simulink model "quadrotor_control2"  (R2017b)
settings: Solver=FixedStepAuto  StartTime=0.0  StopTime=10  FixedStep=0.0001  RelTol=1e-3  EnableMultiTasking=on
PreLoadFcn:
  | m=0;
libraries: simulink x9
settings Model: Creator=GPH_PC  LastModifiedBy=dell
settings DataIOCC: LimitDataPoints=on  SaveFormat=Array
settings OptimizationCC: LifeSpan=inf
settings DebuggingCC: SolverPrmCheckMsg=warning  SFUnexpectedBacktrackingDiag=warning  SFNoUnconditionalDefaultTransitionDiag=warning  SFExecutionAtInitializationDiag=none
settings HardwareCC: ProdBitPerPointer=32  ProdBitPerSizeT=32  ProdBitPerPtrDiffT=32  ProdLargestAtomicFloat=None  ProdIntDivRoundTo=Undefined  ProdEndianess=Unspecified  ProdWordSize=32  ProdHWDeviceType=32-bit Generic
settings ModelReferenceCC: PropagateSignalLabelsOutOfModel=off
settings CodeAppCC: StateflowObjectComments=on
settings GRTTargetCC: TargetLangStandard=C89/C90 (ANSI)  GeneratePreprocessorConditionals=Disable all
settings ConfigComp: CovMetricSettings=dw  CovHtmlReporting=on  CovSaveCumulativeToWorkspaceVar=on  CovSaveSingleToWorkspaceVar=on  CovExternalEMLEnable=off  CovSFcnEnable=off

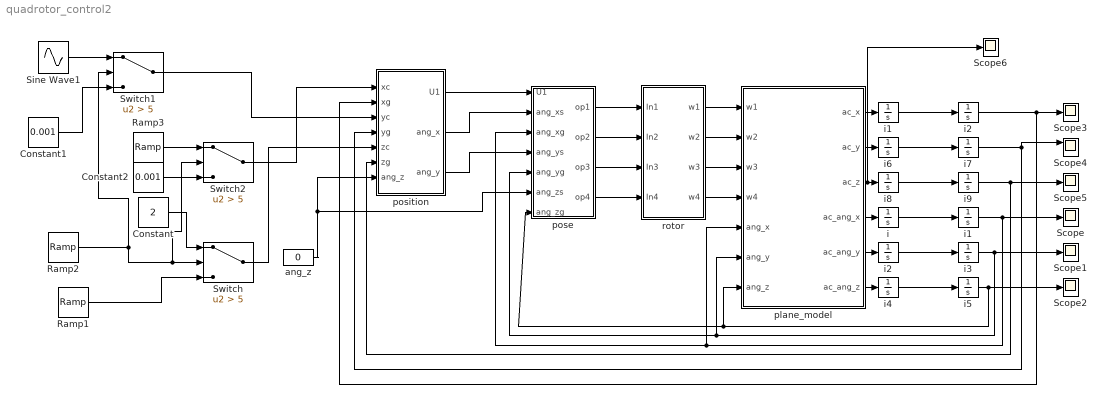
== system quadrotor_control2 ==
  " i1" : Integrator
  " i2" : Integrator
  Constant : Constant  Value=2
  Constant1 : Constant  Value=0.001
  Constant2 : Constant  Value=0.001
  Ramp1 : simulink/Sources/Ramp  slope=0.2  start=0  X0=0
  Ramp2 : simulink/Sources/Ramp  slope=1  start=0  X0=0
  Ramp3 : simulink/Sources/Ramp  slope=1  start=0  X0=0
  Scope{,1..3,5..6} (6 alike) : Scope
  Scope4 : Scope  NumInputPorts=3
  Sine Wave1 : Sin  Amplitude=3  SampleTime=0
  Switch : Switch  Criteria=u2 > Threshold  Threshold=5
  Switch1 : Switch  Criteria=u2 > Threshold  Threshold=5
  Switch2 : Switch  Criteria=u2 > Threshold  Threshold=5
  ang_z : Constant  Value=0
  i{,1..9} (10 alike) : Integrator
  plane_model : MATLAB Function  TreatAsAtomicUnit=on
  pose : Subsystem
  position : Subsystem
  rotor : Subsystem
  wires:
  rotor/1(w1) -> plane_model/1(w1)
  rotor/2(w2) -> plane_model/2(w2)
  rotor/3(w3) -> plane_model/3(w3)
  rotor/4(w4) -> plane_model/4(w4)
  pose/1(op1) -> rotor/1(In1)
  pose/2(op2) -> rotor/2(In2)
  pose/3(op3) -> rotor/3(In3)
  pose/4(op4) -> rotor/4(In4)
  plane_model/4(ac_ang_x) -> i/1
  i/1 -> " i1"/1
  i2/1 -> i3/1
  i4/1 -> i5/1
  plane_model/5(ac_ang_y) -> i2/1
  plane_model/6(ac_ang_z) -> i4/1
  i5/1 -> plane_model/7(ang_z), pose/7(ang_zg), Scope2/1
  i3/1 -> pose/5(ang_yg), plane_model/6(ang_y), Scope1/1
  " i1"/1 -> pose/3(ang_xg), plane_model/5(ang_x), Scope/1
  i1/1 -> " i2"/1
  i6/1 -> i7/1
  i8/1 -> i9/1
  plane_model/3(ac_z) -> Scope6/1, i8/1
  plane_model/2(ac_y) -> i6/1
  plane_model/1(ac_x) -> i1/1
  i9/1 -> Scope5/1, position/6(zg)
  i7/1 -> position/4(yg), Scope4/1
  position/1(U1) -> pose/1(U1)
  position/2(ang_x) -> pose/2(ang_xs)
  position/3(ang_y) -> pose/4(ang_ys)
  ang_z/1 -> position/7(ang_z), pose/6(ang_zs)
  " i2"/1 -> Scope3/1, position/2(xg)
  Constant1/1 -> Switch1/3
  Ramp2/1 -> Switch2/2, Switch/2, Switch1/2
  Constant2/1 -> Switch2/3
  Ramp3/1 -> Switch2/1
  Ramp1/1 -> Switch/3
  Constant/1 -> Switch/1
  Sine Wave1/1 -> Switch1/1
  Switch1/1 -> position/3(yc)
  Switch2/1 -> position/1(xc)
  Switch/1 -> position/5(zc)

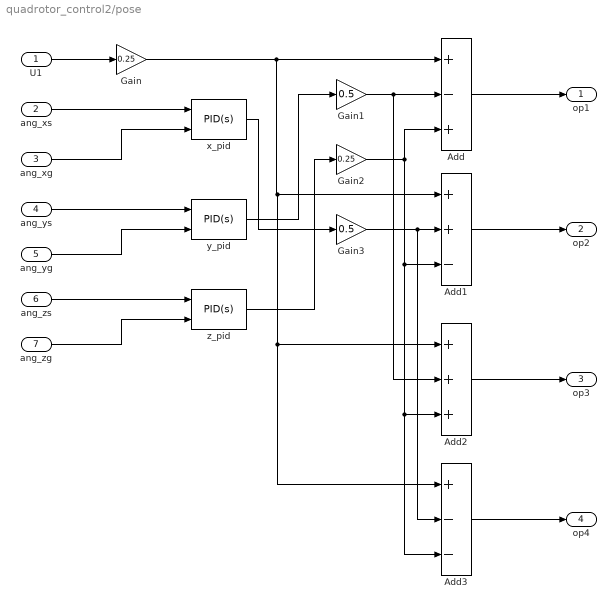
== system quadrotor_control2/pose ==
  U1 : Inport
  ang_xs : Inport  Port=2
  ang_xg : Inport  Port=3
  ang_ys : Inport  Port=4
  ang_yg : Inport  Port=5
  ang_zs : Inport  Port=6
  ang_zg : Inport  Port=7
  Add : Sum  Inputs=+-+
  Add1 : Sum  Inputs=++-
  Add2 : Sum  Inputs=+++
  Add3 : Sum  Inputs=+--
  Gain : Gain  Gain=0.25
  Gain1 : Gain  Gain=0.5
  Gain2 : Gain  Gain=0.25
  Gain3 : Gain  Gain=0.5
  x_pid : simulink/Continuous/PID Controller (2DOF)  Controller=PID  TimeDomain=Continuous-time  SampleTime=-1  IntegratorMethod=Forward Euler  FilterMethod=Forward Euler  Form=Parallel  UseFilter=on  ControllerParametersSource=internal  P=159  I=2  D=90  N=100  b=1  c=1  InitialConditionSource=internal  InitialConditionForIntegrator=0  InitialConditionForFilter=0  ExternalReset=none  LimitOutput=off  UpperSaturationLimit=inf  LowerSaturationLimit=-inf  LinearizeAsGain=on  AntiWindupMode=none  Kb=1  TrackingMode=off  Kt=1  PParamMin=[]  PParamMax=[]  IParamMin=[]  IParamMax=[]  DParamMin=[]  DParamMax=[]  NParamMin=[]  NParamMax=[]  bParamMin=[]  bParamMax=[]  cParamMin=[]  cParamMax=[]  KbParamMin=[]  KbParamMax=[]  KtParamMin=[]  KtParamMax=[]  POutMin=[]  POutMax=[]  IOutMin=[]  IOutMax=[]  DOutMin=[]  DOutMax=[]  NOutMin=[]  NOutMax=[]  bOutMin=[]  bOutMax=[]  cOutMin=[]  cOutMax=[]  KbOutMin=[]  KbOutMax=[]  KtOutMin=[]  KtOutMax=[]  IntegratorOutMin=[]  IntegratorOutMax=[]  FilterOutMin=[]  FilterOutMax=[]  SumOutMin=[]  SumOutMax=[]  Sum1OutMin=[]  Sum1OutMax=[]  Sum2OutMin=[]  Sum2OutMax=[]  Sum3OutMin=[]  Sum3OutMax=[]  SumI1OutMin=[]  SumI1OutMax=[]  SumI2OutMin=[]  SumI2OutMax=[]  SumI3OutMin=[]  SumI3OutMax=[]  SumDOutMin=[]  SumDOutMax=[]  SaturationOutMin=[]  SaturationOutMax=[]  IntegratorContinuousStateAttributes=''  IntegratorStateMustResolveToSignalObject=off  IntegratorRTWStateStorageClass=Auto  FilterContinuousStateAttributes=''  FilterStateMustResolveToSignalObject=off  FilterRTWStateStorageClass=Auto  DifferentiatorICPrevScaledInput=0  DifferentiatorOutMin=[]  DifferentiatorOutMax=[]  InitialConditionSetting=State (most efficient)  FilterDiffOutCoefMin=[]  FilterDiffOutCoefMax=[]  SumDenOutMin=[]  SumDenOutMax=[]  SumNumOutMin=[]  SumNumOutMax=[]  ReciprocalOutMin=[]  ReciprocalOutMax=[]  DivideOutMin=[]  DivideOutMax=[]  TunerSelectOption=Transfer Function Based (PID Tuner App)
  y_pid : simulink/Continuous/PID Controller (2DOF)  Controller=PID  TimeDomain=Continuous-time  SampleTime=-1  IntegratorMethod=Forward Euler  FilterMethod=Forward Euler  Form=Parallel  UseFilter=on  ControllerParametersSource=internal  P=150  I=2  D=90  N=100  b=1  c=1  InitialConditionSource=internal  InitialConditionForIntegrator=0  InitialConditionForFilter=0  ExternalReset=none  LimitOutput=off  UpperSaturationLimit=inf  LowerSaturationLimit=-inf  LinearizeAsGain=on  AntiWindupMode=none  Kb=1  TrackingMode=off  Kt=1  PParamMin=[]  PParamMax=[]  IParamMin=[]  IParamMax=[]  DParamMin=[]  DParamMax=[]  NParamMin=[]  NParamMax=[]  bParamMin=[]  bParamMax=[]  cParamMin=[]  cParamMax=[]  KbParamMin=[]  KbParamMax=[]  KtParamMin=[]  KtParamMax=[]  POutMin=[]  POutMax=[]  IOutMin=[]  IOutMax=[]  DOutMin=[]  DOutMax=[]  NOutMin=[]  NOutMax=[]  bOutMin=[]  bOutMax=[]  cOutMin=[]  cOutMax=[]  KbOutMin=[]  KbOutMax=[]  KtOutMin=[]  KtOutMax=[]  IntegratorOutMin=[]  IntegratorOutMax=[]  FilterOutMin=[]  FilterOutMax=[]  SumOutMin=[]  SumOutMax=[]  Sum1OutMin=[]  Sum1OutMax=[]  Sum2OutMin=[]  Sum2OutMax=[]  Sum3OutMin=[]  Sum3OutMax=[]  SumI1OutMin=[]  SumI1OutMax=[]  SumI2OutMin=[]  SumI2OutMax=[]  SumI3OutMin=[]  SumI3OutMax=[]  SumDOutMin=[]  SumDOutMax=[]  SaturationOutMin=[]  SaturationOutMax=[]  IntegratorContinuousStateAttributes=''  IntegratorStateMustResolveToSignalObject=off  IntegratorRTWStateStorageClass=Auto  FilterContinuousStateAttributes=''  FilterStateMustResolveToSignalObject=off  FilterRTWStateStorageClass=Auto  DifferentiatorICPrevScaledInput=0  DifferentiatorOutMin=[]  DifferentiatorOutMax=[]  InitialConditionSetting=State (most efficient)  FilterDiffOutCoefMin=[]  FilterDiffOutCoefMax=[]  SumDenOutMin=[]  SumDenOutMax=[]  SumNumOutMin=[]  SumNumOutMax=[]  ReciprocalOutMin=[]  ReciprocalOutMax=[]  DivideOutMin=[]  DivideOutMax=[]  TunerSelectOption=Transfer Function Based (PID Tuner App)
  z_pid : simulink/Continuous/PID Controller (2DOF)  Controller=PID  TimeDomain=Continuous-time  SampleTime=-1  IntegratorMethod=Forward Euler  FilterMethod=Forward Euler  Form=Parallel  UseFilter=on  ControllerParametersSource=internal  P=10  I=0  D=20  N=100  b=1  c=1  InitialConditionSource=internal  InitialConditionForIntegrator=0  InitialConditionForFilter=0  ExternalReset=none  LimitOutput=off  UpperSaturationLimit=inf  LowerSaturationLimit=-inf  LinearizeAsGain=on  AntiWindupMode=none  Kb=1  TrackingMode=off  Kt=1  PParamMin=[]  PParamMax=[]  IParamMin=[]  IParamMax=[]  DParamMin=[]  DParamMax=[]  NParamMin=[]  NParamMax=[]  bParamMin=[]  bParamMax=[]  cParamMin=[]  cParamMax=[]  KbParamMin=[]  KbParamMax=[]  KtParamMin=[]  KtParamMax=[]  POutMin=[]  POutMax=[]  IOutMin=[]  IOutMax=[]  DOutMin=[]  DOutMax=[]  NOutMin=[]  NOutMax=[]  bOutMin=[]  bOutMax=[]  cOutMin=[]  cOutMax=[]  KbOutMin=[]  KbOutMax=[]  KtOutMin=[]  KtOutMax=[]  IntegratorOutMin=[]  IntegratorOutMax=[]  FilterOutMin=[]  FilterOutMax=[]  SumOutMin=[]  SumOutMax=[]  Sum1OutMin=[]  Sum1OutMax=[]  Sum2OutMin=[]  Sum2OutMax=[]  Sum3OutMin=[]  Sum3OutMax=[]  SumI1OutMin=[]  SumI1OutMax=[]  SumI2OutMin=[]  SumI2OutMax=[]  SumI3OutMin=[]  SumI3OutMax=[]  SumDOutMin=[]  SumDOutMax=[]  SaturationOutMin=[]  SaturationOutMax=[]  IntegratorContinuousStateAttributes=''  IntegratorStateMustResolveToSignalObject=off  IntegratorRTWStateStorageClass=Auto  FilterContinuousStateAttributes=''  FilterStateMustResolveToSignalObject=off  FilterRTWStateStorageClass=Auto  DifferentiatorICPrevScaledInput=0  DifferentiatorOutMin=[]  DifferentiatorOutMax=[]  InitialConditionSetting=State (most efficient)  FilterDiffOutCoefMin=[]  FilterDiffOutCoefMax=[]  SumDenOutMin=[]  SumDenOutMax=[]  SumNumOutMin=[]  SumNumOutMax=[]  ReciprocalOutMin=[]  ReciprocalOutMax=[]  DivideOutMin=[]  DivideOutMax=[]  TunerSelectOption=Transfer Function Based (PID Tuner App)
  op1 : Outport
  op2 : Outport  Port=2
  op3 : Outport  Port=3
  op4 : Outport  Port=4
  wires:
  Add/1 -> op1/1
  U1/1 -> Gain/1
  Gain/1 -> Add3/1, Add2/1, Add1/1, Add/1
  Gain1/1 -> Add2/2, Add/2
  ang_ys/1 -> y_pid/1
  ang_yg/1 -> y_pid/2
  y_pid/1 -> Gain1/1
  Gain2/1 -> Add/3, Add2/3, Add3/3, Add1/3
  ang_xs/1 -> x_pid/1
  ang_xg/1 -> x_pid/2
  x_pid/1 -> Gain3/1
  Add1/1 -> op2/1
  Gain3/1 -> Add3/2, Add1/2
  ang_zs/1 -> z_pid/1
  ang_zg/1 -> z_pid/2
  z_pid/1 -> Gain2/1
  Add2/1 -> op3/1
  Add3/1 -> op4/1

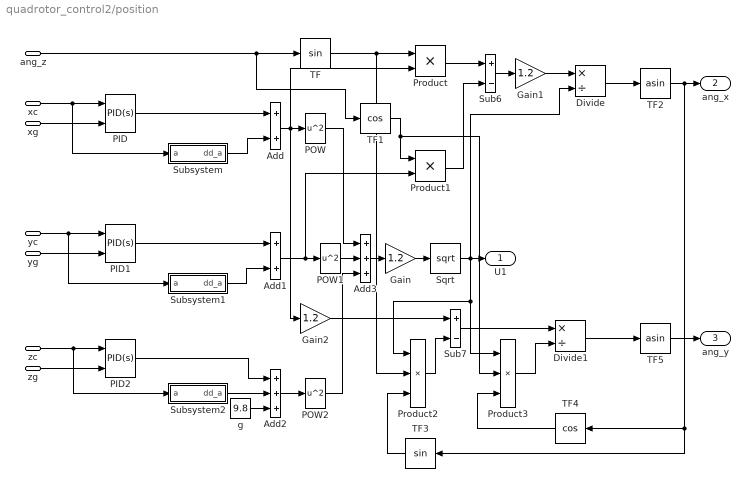
== system quadrotor_control2/position ==
  xc : Inport
  xg : Inport  Port=2
  yc : Inport  Port=3
  yg : Inport  Port=4
  zc : Inport  Port=5
  zg : Inport  Port=6
  ang_z : Inport  Port=7
  Add : Sum
  Add1 : Sum
  Add2 : Sum  Inputs=+++
  Add3 : Sum  Inputs=+++
  Divide : Product  Inputs=*/
  Divide1 : Product  Inputs=*/
  Gain : Gain  Gain=1.2
  Gain1 : Gain  Gain=1.2
  Gain2 : Gain  Gain=1.2
  PID : simulink/Continuous/PID Controller (2DOF)  Controller=PID  TimeDomain=Continuous-time  SampleTime=-1  IntegratorMethod=Forward Euler  FilterMethod=Forward Euler  Form=Parallel  UseFilter=on  ControllerParametersSource=internal  P=70  I=5  D=75  N=100  b=1  c=1  InitialConditionSource=internal  InitialConditionForIntegrator=0  InitialConditionForFilter=0  ExternalReset=none  LimitOutput=off  UpperSaturationLimit=inf  LowerSaturationLimit=-inf  LinearizeAsGain=on  AntiWindupMode=none  Kb=1  TrackingMode=off  Kt=1  PParamMin=[]  PParamMax=[]  IParamMin=[]  IParamMax=[]  DParamMin=[]  DParamMax=[]  NParamMin=[]  NParamMax=[]  bParamMin=[]  bParamMax=[]  cParamMin=[]  cParamMax=[]  KbParamMin=[]  KbParamMax=[]  KtParamMin=[]  KtParamMax=[]  POutMin=[]  POutMax=[]  IOutMin=[]  IOutMax=[]  DOutMin=[]  DOutMax=[]  NOutMin=[]  NOutMax=[]  bOutMin=[]  bOutMax=[]  cOutMin=[]  cOutMax=[]  KbOutMin=[]  KbOutMax=[]  KtOutMin=[]  KtOutMax=[]  IntegratorOutMin=[]  IntegratorOutMax=[]  FilterOutMin=[]  FilterOutMax=[]  SumOutMin=[]  SumOutMax=[]  Sum1OutMin=[]  Sum1OutMax=[]  Sum2OutMin=[]  Sum2OutMax=[]  Sum3OutMin=[]  Sum3OutMax=[]  SumI1OutMin=[]  SumI1OutMax=[]  SumI2OutMin=[]  SumI2OutMax=[]  SumI3OutMin=[]  SumI3OutMax=[]  SumDOutMin=[]  SumDOutMax=[]  SaturationOutMin=[]  SaturationOutMax=[]  IntegratorContinuousStateAttributes=''  IntegratorStateMustResolveToSignalObject=off  IntegratorRTWStateStorageClass=Auto  FilterContinuousStateAttributes=''  FilterStateMustResolveToSignalObject=off  FilterRTWStateStorageClass=Auto  DifferentiatorICPrevScaledInput=0  DifferentiatorOutMin=[]  DifferentiatorOutMax=[]  InitialConditionSetting=State (most efficient)  FilterDiffOutCoefMin=[]  FilterDiffOutCoefMax=[]  SumDenOutMin=[]  SumDenOutMax=[]  SumNumOutMin=[]  SumNumOutMax=[]  ReciprocalOutMin=[]  ReciprocalOutMax=[]  DivideOutMin=[]  DivideOutMax=[]  TunerSelectOption=Transfer Function Based (PID Tuner App)
  PID1 : simulink/Continuous/PID Controller (2DOF)  Controller=PID  TimeDomain=Continuous-time  SampleTime=-1  IntegratorMethod=Forward Euler  FilterMethod=Forward Euler  Form=Parallel  UseFilter=on  ControllerParametersSource=internal  P=75  I=5  D=75  N=100  b=1  c=1  InitialConditionSource=internal  InitialConditionForIntegrator=0  InitialConditionForFilter=0  ExternalReset=none  LimitOutput=off  UpperSaturationLimit=inf  LowerSaturationLimit=-inf  LinearizeAsGain=on  AntiWindupMode=none  Kb=1  TrackingMode=off  Kt=1  PParamMin=[]  PParamMax=[]  IParamMin=[]  IParamMax=[]  DParamMin=[]  DParamMax=[]  NParamMin=[]  NParamMax=[]  bParamMin=[]  bParamMax=[]  cParamMin=[]  cParamMax=[]  KbParamMin=[]  KbParamMax=[]  KtParamMin=[]  KtParamMax=[]  POutMin=[]  POutMax=[]  IOutMin=[]  IOutMax=[]  DOutMin=[]  DOutMax=[]  NOutMin=[]  NOutMax=[]  bOutMin=[]  bOutMax=[]  cOutMin=[]  cOutMax=[]  KbOutMin=[]  KbOutMax=[]  KtOutMin=[]  KtOutMax=[]  IntegratorOutMin=[]  IntegratorOutMax=[]  FilterOutMin=[]  FilterOutMax=[]  SumOutMin=[]  SumOutMax=[]  Sum1OutMin=[]  Sum1OutMax=[]  Sum2OutMin=[]  Sum2OutMax=[]  Sum3OutMin=[]  Sum3OutMax=[]  SumI1OutMin=[]  SumI1OutMax=[]  SumI2OutMin=[]  SumI2OutMax=[]  SumI3OutMin=[]  SumI3OutMax=[]  SumDOutMin=[]  SumDOutMax=[]  SaturationOutMin=[]  SaturationOutMax=[]  IntegratorContinuousStateAttributes=''  IntegratorStateMustResolveToSignalObject=off  IntegratorRTWStateStorageClass=Auto  FilterContinuousStateAttributes=''  FilterStateMustResolveToSignalObject=off  FilterRTWStateStorageClass=Auto  DifferentiatorICPrevScaledInput=0  DifferentiatorOutMin=[]  DifferentiatorOutMax=[]  InitialConditionSetting=State (most efficient)  FilterDiffOutCoefMin=[]  FilterDiffOutCoefMax=[]  SumDenOutMin=[]  SumDenOutMax=[]  SumNumOutMin=[]  SumNumOutMax=[]  ReciprocalOutMin=[]  ReciprocalOutMax=[]  DivideOutMin=[]  DivideOutMax=[]  TunerSelectOption=Transfer Function Based (PID Tuner App)
  PID2 : simulink/Continuous/PID Controller (2DOF)  Controller=PID  TimeDomain=Continuous-time  SampleTime=-1  IntegratorMethod=Forward Euler  FilterMethod=Forward Euler  Form=Parallel  UseFilter=on  ControllerParametersSource=internal  P=200  I=75  D=100  N=100  b=1  c=1  InitialConditionSource=internal  InitialConditionForIntegrator=0  InitialConditionForFilter=0  ExternalReset=none  LimitOutput=off  UpperSaturationLimit=inf  LowerSaturationLimit=-inf  LinearizeAsGain=on  AntiWindupMode=none  Kb=1  TrackingMode=off  Kt=1  PParamMin=[]  PParamMax=[]  IParamMin=[]  IParamMax=[]  DParamMin=[]  DParamMax=[]  NParamMin=[]  NParamMax=[]  bParamMin=[]  bParamMax=[]  cParamMin=[]  cParamMax=[]  KbParamMin=[]  KbParamMax=[]  KtParamMin=[]  KtParamMax=[]  POutMin=[]  POutMax=[]  IOutMin=[]  IOutMax=[]  DOutMin=[]  DOutMax=[]  NOutMin=[]  NOutMax=[]  bOutMin=[]  bOutMax=[]  cOutMin=[]  cOutMax=[]  KbOutMin=[]  KbOutMax=[]  KtOutMin=[]  KtOutMax=[]  IntegratorOutMin=[]  IntegratorOutMax=[]  FilterOutMin=[]  FilterOutMax=[]  SumOutMin=[]  SumOutMax=[]  Sum1OutMin=[]  Sum1OutMax=[]  Sum2OutMin=[]  Sum2OutMax=[]  Sum3OutMin=[]  Sum3OutMax=[]  SumI1OutMin=[]  SumI1OutMax=[]  SumI2OutMin=[]  SumI2OutMax=[]  SumI3OutMin=[]  SumI3OutMax=[]  SumDOutMin=[]  SumDOutMax=[]  SaturationOutMin=[]  SaturationOutMax=[]  IntegratorContinuousStateAttributes=''  IntegratorStateMustResolveToSignalObject=off  IntegratorRTWStateStorageClass=Auto  FilterContinuousStateAttributes=''  FilterStateMustResolveToSignalObject=off  FilterRTWStateStorageClass=Auto  DifferentiatorICPrevScaledInput=0  DifferentiatorOutMin=[]  DifferentiatorOutMax=[]  InitialConditionSetting=State (most efficient)  FilterDiffOutCoefMin=[]  FilterDiffOutCoefMax=[]  SumDenOutMin=[]  SumDenOutMax=[]  SumNumOutMin=[]  SumNumOutMax=[]  ReciprocalOutMin=[]  ReciprocalOutMax=[]  DivideOutMin=[]  DivideOutMax=[]  TunerSelectOption=Transfer Function Based (PID Tuner App)
  POW : Math  Operator=square  SaturateOnIntegerOverflow=on
  POW1 : Math  Operator=square  SaturateOnIntegerOverflow=on
  POW2 : Math  Operator=square  SaturateOnIntegerOverflow=on
  Product : Product
  Product1 : Product
  Product2 : Product  Inputs=3
  Product3 : Product  Inputs=3
  Sqrt : Sqrt  SaturateOnIntegerOverflow=on
  Sub6 : Sum  Inputs=+-
  Sub7 : Sum  Inputs=+-
  Subsystem : Subsystem
  Subsystem1 : Subsystem
  Subsystem2 : Subsystem
  TF : Trigonometry
  TF1 : Trigonometry  Operator=cos
  TF2 : Trigonometry  Operator=asin
  TF3 : Trigonometry
  TF4 : Trigonometry  Operator=cos
  TF5 : Trigonometry  Operator=asin
  g : Constant  Value=9.8
  U1 : Outport
  ang_x : Outport  Port=2
  ang_y : Outport  Port=3
  wires:
  Add/1 -> Gain2/1, Product/2, POW/1
  Add1/1 -> Product1/2, POW1/1
  g/1 -> Add2/3
  Add2/1 -> POW2/1
  POW1/1 -> Add3/2
  POW/1 -> Add3/1
  POW2/1 -> Add3/3
  Add3/1 -> Gain/1
  Gain/1 -> Sqrt/1
  Sqrt/1 -> Product3/1, Product2/1, Divide/2, U1/1
  ang_z/1 -> TF1/1, TF/1
  TF/1 -> Product/1, Product2/2
  Product/1 -> Sub6/1
  TF1/1 -> Product1/1, Product3/2
  Product1/1 -> Sub6/2
  Sub6/1 -> Gain1/1
  Gain1/1 -> Divide/1
  Divide/1 -> TF2/1
  TF2/1 -> TF4/1, TF3/1, ang_x/1
  Gain2/1 -> Sub7/1
  Product2/1 -> Sub7/2
  Sub7/1 -> Divide1/1
  TF3/1 -> Product2/3
  TF4/1 -> Product3/3
  Product3/1 -> Divide1/2
  Divide1/1 -> TF5/1
  TF5/1 -> ang_y/1
  xc/1 -> Subsystem/1(a), PID/1
  xg/1 -> PID/2
  PID/1 -> Add/1
  Subsystem/1(dd_a) -> Add/2
  yc/1 -> Subsystem1/1(a), PID1/1
  yg/1 -> PID1/2
  PID1/1 -> Add1/1
  Subsystem1/1(dd_a) -> Add1/2
  Subsystem2/1(dd_a) -> Add2/2
  PID2/1 -> Add2/1
  zc/1 -> Subsystem2/1(a), PID2/1
  zg/1 -> PID2/2

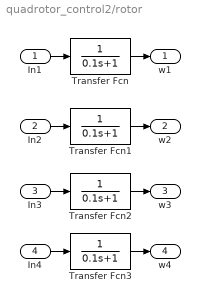
== system quadrotor_control2/rotor ==
  In1 : Inport
  In2 : Inport  Port=2
  In3 : Inport  Port=3
  In4 : Inport  Port=4
  Transfer Fcn{,1..3} (4 alike) : TransferFcn  Denominator=[0.1 1]  AbsoluteTolerance=0.1
  w1 : Outport
  w2 : Outport  Port=2
  w3 : Outport  Port=3
  w4 : Outport  Port=4
  wires:
  Transfer Fcn/1 -> w1/1
  Transfer Fcn3/1 -> w4/1
  In3/1 -> Transfer Fcn2/1
  Transfer Fcn2/1 -> w3/1
  In1/1 -> Transfer Fcn/1
  Transfer Fcn1/1 -> w2/1
  In2/1 -> Transfer Fcn1/1
  In4/1 -> Transfer Fcn3/1

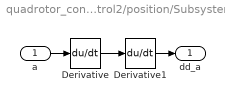
== system quadrotor_control2/position/Subsystem ==
  a : Inport
  Derivative : Derivative
  Derivative1 : Derivative
  dd_a : Outport
  wires:
  Derivative1/1 -> dd_a/1
  a/1 -> Derivative/1
  Derivative/1 -> Derivative1/1

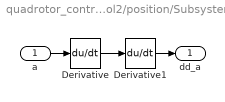
== system quadrotor_control2/position/Subsystem1 ==
  a : Inport
  Derivative : Derivative
  Derivative1 : Derivative
  dd_a : Outport
  wires:
  Derivative1/1 -> dd_a/1
  a/1 -> Derivative/1
  Derivative/1 -> Derivative1/1

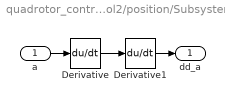
== system quadrotor_control2/position/Subsystem2 ==
  a : Inport
  Derivative : Derivative
  Derivative1 : Derivative
  dd_a : Outport
  wires:
  Derivative1/1 -> dd_a/1
  a/1 -> Derivative/1
  Derivative/1 -> Derivative1/1

== matlab function quadrotor_control2/plane_model ==
  data: w1 input; ac_x output; w2 input; w3 input; w4 input; ac_y output; ac_z output; ac_ang_x output; ac_ang_y output; ac_ang_z output; ang_x input; ang_y input; ang_z input
function [ac_x,ac_y,ac_z,ac_ang_x,ac_ang_y,ac_ang_z] = fcn(w1,w2,w3,w4,ang_x,ang_y,ang_z)
%#codegen
kv=3.1e-5;Ix=17.333;Iy=17.33;Iz=4.33;m=1.2;
U1=kv*(w1*w1+w2*w2+w3*w3+w4*w4);
U2=kv*(w2*w2-w4*w4);
U3=kv*(w3*w3-w1*w1);
U4=kv*(w1*w1+w3*w3-w2*w2-w4*w4);
ac_x=U1*(sin(ang_x)*sin(ang_z)+cos(ang_z)*sin(ang_y)*cos(ang_x))/m;
ac_y=U1*(sin(ang_z)*sin(ang_y)*cos(ang_x)-cos(ang_z)*sin(ang_x))/m;
ac_z=U1*cos(ang_x)*cos(ang_y)/m-9.8;
ac_ang_x=U2*Ix;
ac_ang_y=U3*Iy; 
ac_ang_z=U4*Iz;
